simulink model "ModID_b2_R2018A1_withCF"  (R2018a)
settings: Solver=VariableStepAuto  StartTime=0.0  StopTime=10.0  RelTol=1e-3
undefined symbols (not defined in the file or in its folder): par
settings Model: Creator=janneke  LastModifiedBy=jessi
settings SolverCC: ZeroCrossAlgorithm=Adaptive
settings DebuggingCC: MaxConsecutiveZCsMsg=none  LibraryContextMissingDiagnostic=warning
settings SFSimCC: SimUseLocalCustomCode=on
settings RTWCC: RTWUseLocalCustomCode=on

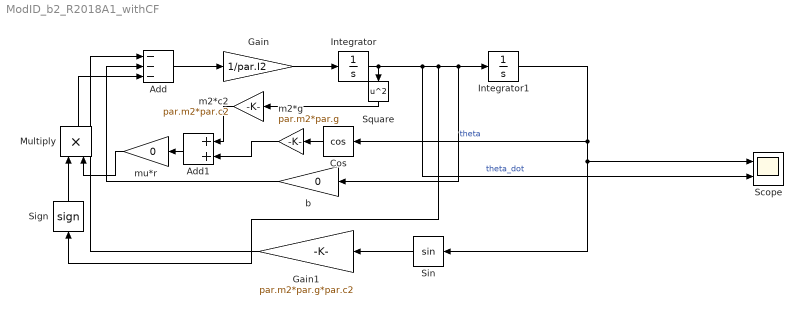
== system ModID_b2_R2018A1_withCF ==
  Add : Sum  Inputs=---
  Add1 : Sum
  Cos : Trigonometry  Operator=cos
  Gain : Gain  Gain=1/par.I2
  Gain1 : Gain  Gain=par.m2*par.g*par.c2
  Integrator : Integrator
  Integrator1 : Integrator  InitialCondition=-pi/2
  Multiply : Product
  Scope : Scope  NumInputPorts=2
  Sign : Signum
  Sin : Trigonometry
  Square : Math  Operator=square  SaturateOnIntegerOverflow=on
  b : Gain  Gain=0
  m2*c2 : Gain  Gain=par.m2*par.c2
  m2*g : Gain  Gain=par.m2*par.g
  "mu*r " : Gain  Gain=0
  wires:
  Integrator/1 -> Scope/2, Sign/1, b/1, Integrator1/1, Square/1  "theta_dot"
  Integrator1/1 -> Sin/1, Scope/1, Cos/1  "theta"
  Gain/1 -> Integrator/1
  Add/1 -> Gain/1
  Sin/1 -> Gain1/1
  Gain1/1 -> Add/1
  b/1 -> Add/2
  Add1/1 -> "mu*r "/1
  m2*c2/1 -> Add1/1
  Square/1 -> m2*c2/1
  m2*g/1 -> Add1/2
  Cos/1 -> m2*g/1
  Sign/1 -> Multiply/1
  "mu*r "/1 -> Multiply/2
  Multiply/1 -> Add/3
